simulink model "step4_BatteryModel"  (R2026a)
settings: Solver=daessc  StopTime=82524.31  FixedStep=1e-2  MaxStep=10  MinStep=1e-2  AbsTol=1e-4
undefined symbols (not defined in the file or in its folder): battery_builder_rtmsupport, gcbh
libraries: SHP320_Batteries_lib x8, fl_lib x3, nesl_utility x3, batt_lib x2
(part 2 of 2)

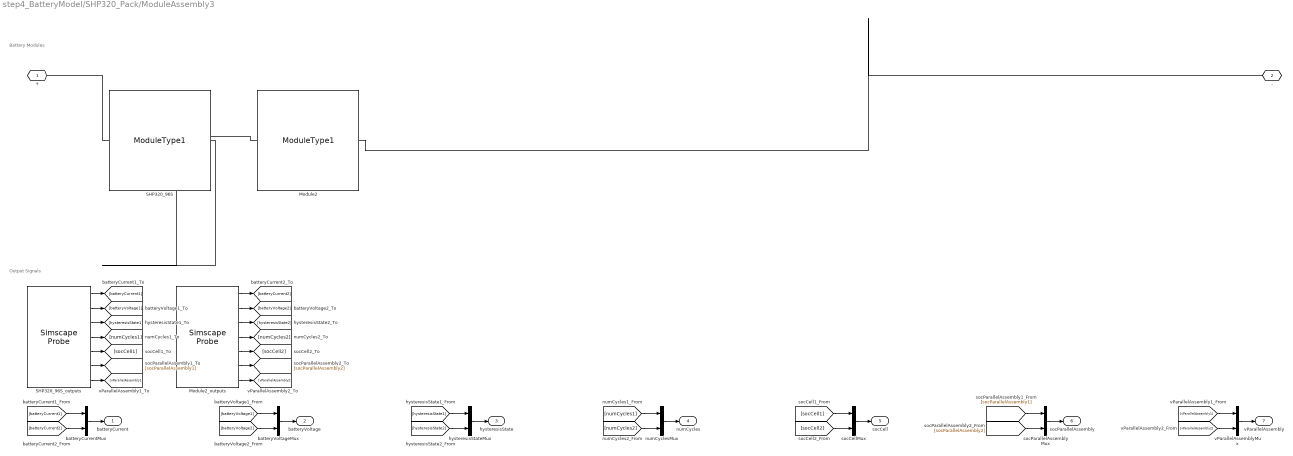
== system step4_BatteryModel/SHP320_Pack/ModuleAssembly3 ==
  note: Output Signals
  note: Battery Modules
  Module2 : SHP320_Batteries_lib/Modules/ModuleType1  BatteryCapacityCell=ModuleType1.BatteryCapacityCell A*hr  ExtrapolationMethodCell=simscape.enum.extrapolation.nearest  SOCBreakpointsCell=ModuleType1.SOCBreakpointsCell  TemperatureBreakpointsCell=ModuleType1.TemperatureBreakpointsCell K  OpenCircuitVoltageThermalCell=ModuleType1.OpenCircuitVoltageThermalCell V  VoltageRangeCell=ModuleType1.VoltageRangeCell V  MaximumHysteresisVoltageThermalCell=ModuleType1.MaximumHysteresisVoltageThermalCell V  InstantaneousHysteresisVoltageThermalCell=ModuleType1.InstantaneousHysteresisVoltageThermalCell V  HysteresisRateThermalCell=ModuleType1.HysteresisRateThermalCell  ResistanceSOCBreakpointsCell=ModuleType1.ResistanceSOCBreakpointsCell  ResistanceTemperatureBreakpointsCell=ModuleType1.ResistanceTemperatureBreakpointsCell K  ChargeR0ThermalCell=ModuleType1.ChargeR0ThermalCell Ohm  DischargeR0ThermalCell=ModuleType1.DischargeR0ThermalCell Ohm  DischargeR1ThermalCell=ModuleType1.DischargeR1ThermalCell Ohm  DischargeTau1ThermalCell=ModuleType1.DischargeTau1ThermalCell s  ChargeR1ThermalCell=ModuleType1.ChargeR1ThermalCell Ohm  ChargeTau1ThermalCell=ModuleType1.ChargeTau1ThermalCell s  DischargeR2ThermalCell=ModuleType1.DischargeR2ThermalCell Ohm  DischargeTau2ThermalCell=ModuleType1.DischargeTau2ThermalCell s  ChargeR2ThermalCell=ModuleType1.ChargeR2ThermalCell Ohm  ChargeTau2ThermalCell=ModuleType1.ChargeTau2ThermalCell s  SimulationTemperatureCell=ModuleType1.SimulationTemperatureCell K  socCell_specify=on  socCell_priority=High  socCell=ModuleAssembly3.Module2.socCell  socCell_nominal_specify=off  socCell_nominal_value=1  socCell_nominal_unit=1  batteryVoltage_specify=on  batteryVoltage_priority=None  batteryVoltage=ModuleAssembly3.Module2.batteryVoltage V  batteryVoltage_nominal_specify=off  batteryVoltage_nominal_value=1  batteryVoltage_nominal_unit=V  batteryCurrent_specify=on  batteryCurrent_priority=None  batteryCurrent=ModuleAssembly3.Module2.batteryCurrent A  batteryCurrent_nominal_specify=off  batteryCurrent_nominal_value=1  batteryCurrent_nominal_unit=A  numCycles_specify=on  numCycles_priority=High  numCycles=ModuleAssembly3.Module2.numCycles  numCycles_nominal_specify=off  numCycles_nominal_value=1  numCycles_nominal_unit=1  hysteresisState_specify=on  hysteresisState_priority=High  hysteresisState=ModuleAssembly3.Module2.hysteresisState  hysteresisState_nominal_specify=off  hysteresisState_nominal_value=1  hysteresisState_nominal_unit=1  vParallelAssembly_specify=on  vParallelAssembly_priority=None  vParallelAssembly=ModuleAssembly3.Module2.vParallelAssembly V  vParallelAssembly_nominal_specify=off  vParallelAssembly_nominal_value=1  vParallelAssembly_nominal_unit=V  socParallelAssembly_specify=on  socParallelAssembly_priority=None  socParallelAssembly=ModuleAssembly3.Module2.socParallelAssembly  socParallelAssembly_nominal_specify=off  socParallelAssembly_nominal_value=1  socParallelAssembly_nominal_unit=1
  Module2_outputs : SimscapeProbe  BoundBlock=72  Variables="{\"batteryCurrent\":{\"Probing\":\"ON\"},\"batteryVoltage\":{\"Probing\":\"ON\"},\"hysteresisState\":{\"Probing\":\"ON\"},\"numCycles\":{\"Probing\":\"ON\"},\"socCell\":{\"Probing\":\"ON\"},\"socParallelAssembly\":{\"Probing\":\"ON\"},\"vParallelAssembly\":{\"Probing\":\"ON\"}}"
  SHP320_96S : SHP320_Batteries_lib/Modules/ModuleType1  BatteryCapacityCell=ModuleType1.BatteryCapacityCell A*hr  ExtrapolationMethodCell=simscape.enum.extrapolation.nearest  SOCBreakpointsCell=ModuleType1.SOCBreakpointsCell  TemperatureBreakpointsCell=ModuleType1.TemperatureBreakpointsCell K  OpenCircuitVoltageThermalCell=ModuleType1.OpenCircuitVoltageThermalCell V  VoltageRangeCell=ModuleType1.VoltageRangeCell V  MaximumHysteresisVoltageThermalCell=ModuleType1.MaximumHysteresisVoltageThermalCell V  InstantaneousHysteresisVoltageThermalCell=ModuleType1.InstantaneousHysteresisVoltageThermalCell V  HysteresisRateThermalCell=ModuleType1.HysteresisRateThermalCell  ResistanceSOCBreakpointsCell=ModuleType1.ResistanceSOCBreakpointsCell  ResistanceTemperatureBreakpointsCell=ModuleType1.ResistanceTemperatureBreakpointsCell K  ChargeR0ThermalCell=ModuleType1.ChargeR0ThermalCell Ohm  DischargeR0ThermalCell=ModuleType1.DischargeR0ThermalCell Ohm  DischargeR1ThermalCell=ModuleType1.DischargeR1ThermalCell Ohm  DischargeTau1ThermalCell=ModuleType1.DischargeTau1ThermalCell s  ChargeR1ThermalCell=ModuleType1.ChargeR1ThermalCell Ohm  ChargeTau1ThermalCell=ModuleType1.ChargeTau1ThermalCell s  DischargeR2ThermalCell=ModuleType1.DischargeR2ThermalCell Ohm  DischargeTau2ThermalCell=ModuleType1.DischargeTau2ThermalCell s  ChargeR2ThermalCell=ModuleType1.ChargeR2ThermalCell Ohm  ChargeTau2ThermalCell=ModuleType1.ChargeTau2ThermalCell s  SimulationTemperatureCell=ModuleType1.SimulationTemperatureCell K  socCell_specify=on  socCell_priority=High  socCell=ModuleAssembly3.SHP320_96S.socCell  socCell_nominal_specify=off  socCell_nominal_value=1  socCell_nominal_unit=1  batteryVoltage_specify=on  batteryVoltage_priority=None  batteryVoltage=ModuleAssembly3.SHP320_96S.batteryVoltage V  batteryVoltage_nominal_specify=off  batteryVoltage_nominal_value=1  batteryVoltage_nominal_unit=V  batteryCurrent_specify=on  batteryCurrent_priority=None  batteryCurrent=ModuleAssembly3.SHP320_96S.batteryCurrent A  batteryCurrent_nominal_specify=off  batteryCurrent_nominal_value=1  batteryCurrent_nominal_unit=A  numCycles_specify=on  numCycles_priority=High  numCycles=ModuleAssembly3.SHP320_96S.numCycles  numCycles_nominal_specify=off  numCycles_nominal_value=1  numCycles_nominal_unit=1  hysteresisState_specify=on  hysteresisState_priority=High  hysteresisState=ModuleAssembly3.SHP320_96S.hysteresisState  hysteresisState_nominal_specify=off  hysteresisState_nominal_value=1  hysteresisState_nominal_unit=1  vParallelAssembly_specify=on  vParallelAssembly_priority=None  vParallelAssembly=ModuleAssembly3.SHP320_96S.vParallelAssembly V  vParallelAssembly_nominal_specify=off  vParallelAssembly_nominal_value=1  vParallelAssembly_nominal_unit=V  socParallelAssembly_specify=on  socParallelAssembly_priority=None  socParallelAssembly=ModuleAssembly3.SHP320_96S.socParallelAssembly  socParallelAssembly_nominal_specify=off  socParallelAssembly_nominal_value=1  socParallelAssembly_nominal_unit=1
  SHP320_96S_outputs : SimscapeProbe  BoundBlock=74  Variables="{\"batteryCurrent\":{\"Probing\":\"ON\"},\"batteryVoltage\":{\"Probing\":\"ON\"},\"hysteresisState\":{\"Probing\":\"ON\"},\"numCycles\":{\"Probing\":\"ON\"},\"socCell\":{\"Probing\":\"ON\"},\"socParallelAssembly\":{\"Probing\":\"ON\"},\"vParallelAssembly\":{\"Probing\":\"ON\"}}"
  batteryCurrentMux : Mux  Inputs=2
  batteryVoltageMux : Mux  Inputs=2
  hysteresisStateMux : Mux  Inputs=2
  numCyclesMux : Mux  Inputs=2
  socCellMux : Mux  Inputs=2
  socParallelAssemblyMux : Mux  Inputs=2
  vParallelAssemblyMux : Mux  Inputs=2
  + : PMIOPort  Side=Left
  - : PMIOPort  Port=2  Side=Right
  batteryCurrent : Outport
  batteryVoltage : Outport  Port=2
  hysteresisState : Outport  Port=3
  numCycles : Outport  Port=4
  socCell : Outport  Port=5
  socParallelAssembly : Outport  Port=6
  vParallelAssembly : Outport  Port=7
  wires:
  [vParallelAssembly2] -> vParallelAssemblyMux/2
  Module2_outputs/7 -> [vParallelAssembly2]
  [socParallelAssembly2] -> socParallelAssemblyMux/2
  Module2_outputs/6 -> [socParallelAssembly2]
  [socCell2] -> socCellMux/2
  Module2_outputs/5 -> [socCell2]
  [numCycles2] -> numCyclesMux/2
  Module2_outputs/4 -> [numCycles2]
  [hysteresisState2] -> hysteresisStateMux/2
  Module2_outputs/3 -> [hysteresisState2]
  [batteryVoltage2] -> batteryVoltageMux/2
  Module2_outputs/2 -> [batteryVoltage2]
  [batteryCurrent2] -> batteryCurrentMux/2
  Module2_outputs/1 -> [batteryCurrent2]
  [vParallelAssembly1] -> vParallelAssemblyMux/1
  vParallelAssemblyMux/1 -> vParallelAssembly/1
  SHP320_96S_outputs/7 -> [vParallelAssembly1]
  [socParallelAssembly1] -> socParallelAssemblyMux/1
  socParallelAssemblyMux/1 -> socParallelAssembly/1
  SHP320_96S_outputs/6 -> [socParallelAssembly1]
  [socCell1] -> socCellMux/1
  socCellMux/1 -> socCell/1
  SHP320_96S_outputs/5 -> [socCell1]
  [numCycles1] -> numCyclesMux/1
  numCyclesMux/1 -> numCycles/1
  SHP320_96S_outputs/4 -> [numCycles1]
  [hysteresisState1] -> hysteresisStateMux/1
  hysteresisStateMux/1 -> hysteresisState/1
  SHP320_96S_outputs/3 -> [hysteresisState1]
  [batteryVoltage1] -> batteryVoltageMux/1
  batteryVoltageMux/1 -> batteryVoltage/1
  SHP320_96S_outputs/2 -> [batteryVoltage1]
  [batteryCurrent1] -> batteryCurrentMux/1
  batteryCurrentMux/1 -> batteryCurrent/1
  SHP320_96S_outputs/1 -> [batteryCurrent1]
  connections:
  Module2/RConn1 -- -/RConn1
  SHP320_96S/LConn1 -- +/RConn1
  Module2/LConn1 -- SHP320_96S/RConn1

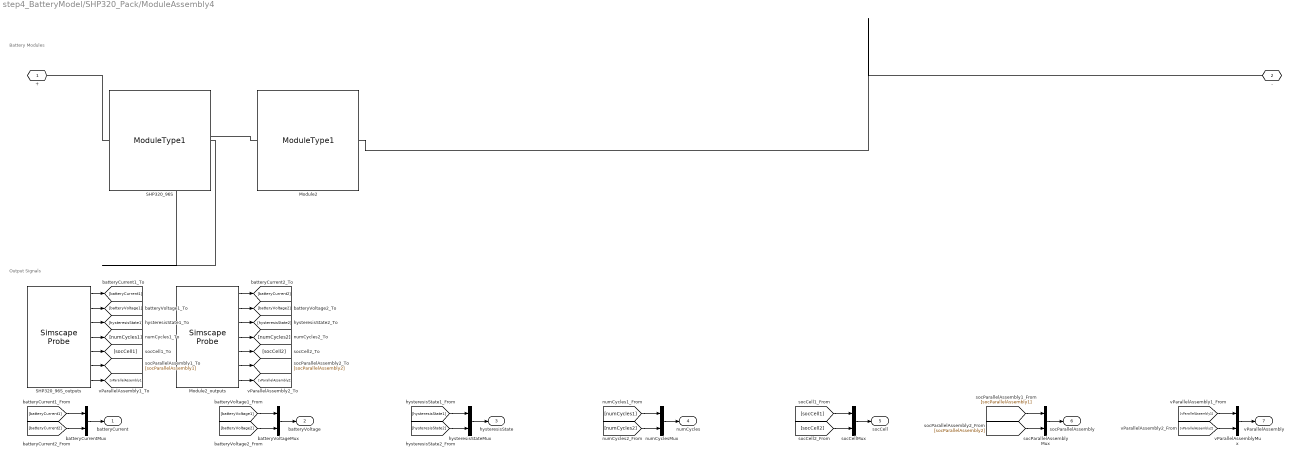
== system step4_BatteryModel/SHP320_Pack/ModuleAssembly4 ==
  note: Output Signals
  note: Battery Modules
  Module2 : SHP320_Batteries_lib/Modules/ModuleType1  BatteryCapacityCell=ModuleType1.BatteryCapacityCell A*hr  ExtrapolationMethodCell=simscape.enum.extrapolation.nearest  SOCBreakpointsCell=ModuleType1.SOCBreakpointsCell  TemperatureBreakpointsCell=ModuleType1.TemperatureBreakpointsCell K  OpenCircuitVoltageThermalCell=ModuleType1.OpenCircuitVoltageThermalCell V  VoltageRangeCell=ModuleType1.VoltageRangeCell V  MaximumHysteresisVoltageThermalCell=ModuleType1.MaximumHysteresisVoltageThermalCell V  InstantaneousHysteresisVoltageThermalCell=ModuleType1.InstantaneousHysteresisVoltageThermalCell V  HysteresisRateThermalCell=ModuleType1.HysteresisRateThermalCell  ResistanceSOCBreakpointsCell=ModuleType1.ResistanceSOCBreakpointsCell  ResistanceTemperatureBreakpointsCell=ModuleType1.ResistanceTemperatureBreakpointsCell K  ChargeR0ThermalCell=ModuleType1.ChargeR0ThermalCell Ohm  DischargeR0ThermalCell=ModuleType1.DischargeR0ThermalCell Ohm  DischargeR1ThermalCell=ModuleType1.DischargeR1ThermalCell Ohm  DischargeTau1ThermalCell=ModuleType1.DischargeTau1ThermalCell s  ChargeR1ThermalCell=ModuleType1.ChargeR1ThermalCell Ohm  ChargeTau1ThermalCell=ModuleType1.ChargeTau1ThermalCell s  DischargeR2ThermalCell=ModuleType1.DischargeR2ThermalCell Ohm  DischargeTau2ThermalCell=ModuleType1.DischargeTau2ThermalCell s  ChargeR2ThermalCell=ModuleType1.ChargeR2ThermalCell Ohm  ChargeTau2ThermalCell=ModuleType1.ChargeTau2ThermalCell s  SimulationTemperatureCell=ModuleType1.SimulationTemperatureCell K  socCell_specify=on  socCell_priority=High  socCell=ModuleAssembly4.Module2.socCell  socCell_nominal_specify=off  socCell_nominal_value=1  socCell_nominal_unit=1  batteryVoltage_specify=on  batteryVoltage_priority=None  batteryVoltage=ModuleAssembly4.Module2.batteryVoltage V  batteryVoltage_nominal_specify=off  batteryVoltage_nominal_value=1  batteryVoltage_nominal_unit=V  batteryCurrent_specify=on  batteryCurrent_priority=None  batteryCurrent=ModuleAssembly4.Module2.batteryCurrent A  batteryCurrent_nominal_specify=off  batteryCurrent_nominal_value=1  batteryCurrent_nominal_unit=A  numCycles_specify=on  numCycles_priority=High  numCycles=ModuleAssembly4.Module2.numCycles  numCycles_nominal_specify=off  numCycles_nominal_value=1  numCycles_nominal_unit=1  hysteresisState_specify=on  hysteresisState_priority=High  hysteresisState=ModuleAssembly4.Module2.hysteresisState  hysteresisState_nominal_specify=off  hysteresisState_nominal_value=1  hysteresisState_nominal_unit=1  vParallelAssembly_specify=on  vParallelAssembly_priority=None  vParallelAssembly=ModuleAssembly4.Module2.vParallelAssembly V  vParallelAssembly_nominal_specify=off  vParallelAssembly_nominal_value=1  vParallelAssembly_nominal_unit=V  socParallelAssembly_specify=on  socParallelAssembly_priority=None  socParallelAssembly=ModuleAssembly4.Module2.socParallelAssembly  socParallelAssembly_nominal_specify=off  socParallelAssembly_nominal_value=1  socParallelAssembly_nominal_unit=1
  Module2_outputs : SimscapeProbe  BoundBlock=123  Variables="{\"batteryCurrent\":{\"Probing\":\"ON\"},\"batteryVoltage\":{\"Probing\":\"ON\"},\"hysteresisState\":{\"Probing\":\"ON\"},\"numCycles\":{\"Probing\":\"ON\"},\"socCell\":{\"Probing\":\"ON\"},\"socParallelAssembly\":{\"Probing\":\"ON\"},\"vParallelAssembly\":{\"Probing\":\"ON\"}}"
  SHP320_96S : SHP320_Batteries_lib/Modules/ModuleType1  BatteryCapacityCell=ModuleType1.BatteryCapacityCell A*hr  ExtrapolationMethodCell=simscape.enum.extrapolation.nearest  SOCBreakpointsCell=ModuleType1.SOCBreakpointsCell  TemperatureBreakpointsCell=ModuleType1.TemperatureBreakpointsCell K  OpenCircuitVoltageThermalCell=ModuleType1.OpenCircuitVoltageThermalCell V  VoltageRangeCell=ModuleType1.VoltageRangeCell V  MaximumHysteresisVoltageThermalCell=ModuleType1.MaximumHysteresisVoltageThermalCell V  InstantaneousHysteresisVoltageThermalCell=ModuleType1.InstantaneousHysteresisVoltageThermalCell V  HysteresisRateThermalCell=ModuleType1.HysteresisRateThermalCell  ResistanceSOCBreakpointsCell=ModuleType1.ResistanceSOCBreakpointsCell  ResistanceTemperatureBreakpointsCell=ModuleType1.ResistanceTemperatureBreakpointsCell K  ChargeR0ThermalCell=ModuleType1.ChargeR0ThermalCell Ohm  DischargeR0ThermalCell=ModuleType1.DischargeR0ThermalCell Ohm  DischargeR1ThermalCell=ModuleType1.DischargeR1ThermalCell Ohm  DischargeTau1ThermalCell=ModuleType1.DischargeTau1ThermalCell s  ChargeR1ThermalCell=ModuleType1.ChargeR1ThermalCell Ohm  ChargeTau1ThermalCell=ModuleType1.ChargeTau1ThermalCell s  DischargeR2ThermalCell=ModuleType1.DischargeR2ThermalCell Ohm  DischargeTau2ThermalCell=ModuleType1.DischargeTau2ThermalCell s  ChargeR2ThermalCell=ModuleType1.ChargeR2ThermalCell Ohm  ChargeTau2ThermalCell=ModuleType1.ChargeTau2ThermalCell s  SimulationTemperatureCell=ModuleType1.SimulationTemperatureCell K  socCell_specify=on  socCell_priority=High  socCell=ModuleAssembly4.SHP320_96S.socCell  socCell_nominal_specify=off  socCell_nominal_value=1  socCell_nominal_unit=1  batteryVoltage_specify=on  batteryVoltage_priority=None  batteryVoltage=ModuleAssembly4.SHP320_96S.batteryVoltage V  batteryVoltage_nominal_specify=off  batteryVoltage_nominal_value=1  batteryVoltage_nominal_unit=V  batteryCurrent_specify=on  batteryCurrent_priority=None  batteryCurrent=ModuleAssembly4.SHP320_96S.batteryCurrent A  batteryCurrent_nominal_specify=off  batteryCurrent_nominal_value=1  batteryCurrent_nominal_unit=A  numCycles_specify=on  numCycles_priority=High  numCycles=ModuleAssembly4.SHP320_96S.numCycles  numCycles_nominal_specify=off  numCycles_nominal_value=1  numCycles_nominal_unit=1  hysteresisState_specify=on  hysteresisState_priority=High  hysteresisState=ModuleAssembly4.SHP320_96S.hysteresisState  hysteresisState_nominal_specify=off  hysteresisState_nominal_value=1  hysteresisState_nominal_unit=1  vParallelAssembly_specify=on  vParallelAssembly_priority=None  vParallelAssembly=ModuleAssembly4.SHP320_96S.vParallelAssembly V  vParallelAssembly_nominal_specify=off  vParallelAssembly_nominal_value=1  vParallelAssembly_nominal_unit=V  socParallelAssembly_specify=on  socParallelAssembly_priority=None  socParallelAssembly=ModuleAssembly4.SHP320_96S.socParallelAssembly  socParallelAssembly_nominal_specify=off  socParallelAssembly_nominal_value=1  socParallelAssembly_nominal_unit=1
  SHP320_96S_outputs : SimscapeProbe  BoundBlock=125  Variables="{\"batteryCurrent\":{\"Probing\":\"ON\"},\"batteryVoltage\":{\"Probing\":\"ON\"},\"hysteresisState\":{\"Probing\":\"ON\"},\"numCycles\":{\"Probing\":\"ON\"},\"socCell\":{\"Probing\":\"ON\"},\"socParallelAssembly\":{\"Probing\":\"ON\"},\"vParallelAssembly\":{\"Probing\":\"ON\"}}"
  batteryCurrentMux : Mux  Inputs=2
  batteryVoltageMux : Mux  Inputs=2
  hysteresisStateMux : Mux  Inputs=2
  numCyclesMux : Mux  Inputs=2
  socCellMux : Mux  Inputs=2
  socParallelAssemblyMux : Mux  Inputs=2
  vParallelAssemblyMux : Mux  Inputs=2
  + : PMIOPort  Side=Left
  - : PMIOPort  Port=2  Side=Right
  batteryCurrent : Outport
  batteryVoltage : Outport  Port=2
  hysteresisState : Outport  Port=3
  numCycles : Outport  Port=4
  socCell : Outport  Port=5
  socParallelAssembly : Outport  Port=6
  vParallelAssembly : Outport  Port=7
  wires:
  [vParallelAssembly2] -> vParallelAssemblyMux/2
  Module2_outputs/7 -> [vParallelAssembly2]
  [socParallelAssembly2] -> socParallelAssemblyMux/2
  Module2_outputs/6 -> [socParallelAssembly2]
  [socCell2] -> socCellMux/2
  Module2_outputs/5 -> [socCell2]
  [numCycles2] -> numCyclesMux/2
  Module2_outputs/4 -> [numCycles2]
  [hysteresisState2] -> hysteresisStateMux/2
  Module2_outputs/3 -> [hysteresisState2]
  [batteryVoltage2] -> batteryVoltageMux/2
  Module2_outputs/2 -> [batteryVoltage2]
  [batteryCurrent2] -> batteryCurrentMux/2
  Module2_outputs/1 -> [batteryCurrent2]
  [vParallelAssembly1] -> vParallelAssemblyMux/1
  vParallelAssemblyMux/1 -> vParallelAssembly/1
  SHP320_96S_outputs/7 -> [vParallelAssembly1]
  [socParallelAssembly1] -> socParallelAssemblyMux/1
  socParallelAssemblyMux/1 -> socParallelAssembly/1
  SHP320_96S_outputs/6 -> [socParallelAssembly1]
  [socCell1] -> socCellMux/1
  socCellMux/1 -> socCell/1
  SHP320_96S_outputs/5 -> [socCell1]
  [numCycles1] -> numCyclesMux/1
  numCyclesMux/1 -> numCycles/1
  SHP320_96S_outputs/4 -> [numCycles1]
  [hysteresisState1] -> hysteresisStateMux/1
  hysteresisStateMux/1 -> hysteresisState/1
  SHP320_96S_outputs/3 -> [hysteresisState1]
  [batteryVoltage1] -> batteryVoltageMux/1
  batteryVoltageMux/1 -> batteryVoltage/1
  SHP320_96S_outputs/2 -> [batteryVoltage1]
  [batteryCurrent1] -> batteryCurrentMux/1
  batteryCurrentMux/1 -> batteryCurrent/1
  SHP320_96S_outputs/1 -> [batteryCurrent1]
  connections:
  Module2/RConn1 -- -/RConn1
  SHP320_96S/LConn1 -- +/RConn1
  Module2/LConn1 -- SHP320_96S/RConn1

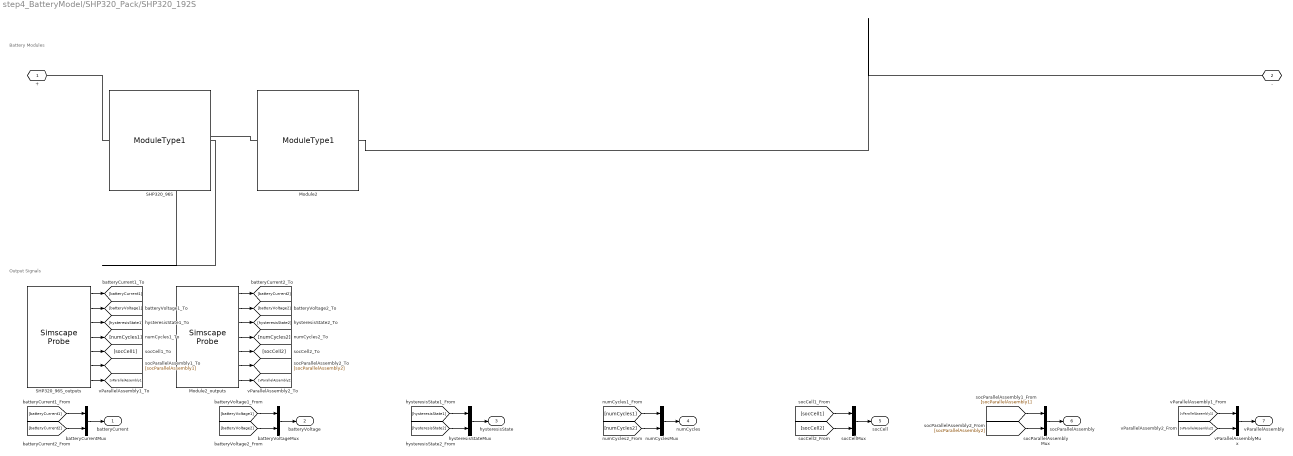
== system step4_BatteryModel/SHP320_Pack/SHP320_192S ==
  note: Output Signals
  note: Battery Modules
  Module2 : SHP320_Batteries_lib/Modules/ModuleType1  BatteryCapacityCell=ModuleType1.BatteryCapacityCell A*hr  ExtrapolationMethodCell=simscape.enum.extrapolation.nearest  SOCBreakpointsCell=ModuleType1.SOCBreakpointsCell  TemperatureBreakpointsCell=ModuleType1.TemperatureBreakpointsCell K  OpenCircuitVoltageThermalCell=ModuleType1.OpenCircuitVoltageThermalCell V  VoltageRangeCell=ModuleType1.VoltageRangeCell V  MaximumHysteresisVoltageThermalCell=ModuleType1.MaximumHysteresisVoltageThermalCell V  InstantaneousHysteresisVoltageThermalCell=ModuleType1.InstantaneousHysteresisVoltageThermalCell V  HysteresisRateThermalCell=ModuleType1.HysteresisRateThermalCell  ResistanceSOCBreakpointsCell=ModuleType1.ResistanceSOCBreakpointsCell  ResistanceTemperatureBreakpointsCell=ModuleType1.ResistanceTemperatureBreakpointsCell K  ChargeR0ThermalCell=ModuleType1.ChargeR0ThermalCell Ohm  DischargeR0ThermalCell=ModuleType1.DischargeR0ThermalCell Ohm  DischargeR1ThermalCell=ModuleType1.DischargeR1ThermalCell Ohm  DischargeTau1ThermalCell=ModuleType1.DischargeTau1ThermalCell s  ChargeR1ThermalCell=ModuleType1.ChargeR1ThermalCell Ohm  ChargeTau1ThermalCell=ModuleType1.ChargeTau1ThermalCell s  DischargeR2ThermalCell=ModuleType1.DischargeR2ThermalCell Ohm  DischargeTau2ThermalCell=ModuleType1.DischargeTau2ThermalCell s  ChargeR2ThermalCell=ModuleType1.ChargeR2ThermalCell Ohm  ChargeTau2ThermalCell=ModuleType1.ChargeTau2ThermalCell s  SimulationTemperatureCell=ModuleType1.SimulationTemperatureCell K  socCell_specify=on  socCell_priority=High  socCell=SHP320_192S.Module2.socCell  socCell_nominal_specify=off  socCell_nominal_value=1  socCell_nominal_unit=1  batteryVoltage_specify=on  batteryVoltage_priority=None  batteryVoltage=SHP320_192S.Module2.batteryVoltage V  batteryVoltage_nominal_specify=off  batteryVoltage_nominal_value=1  batteryVoltage_nominal_unit=V  batteryCurrent_specify=on  batteryCurrent_priority=None  batteryCurrent=SHP320_192S.Module2.batteryCurrent A  batteryCurrent_nominal_specify=off  batteryCurrent_nominal_value=1  batteryCurrent_nominal_unit=A  numCycles_specify=on  numCycles_priority=High  numCycles=SHP320_192S.Module2.numCycles  numCycles_nominal_specify=off  numCycles_nominal_value=1  numCycles_nominal_unit=1  hysteresisState_specify=on  hysteresisState_priority=High  hysteresisState=SHP320_192S.Module2.hysteresisState  hysteresisState_nominal_specify=off  hysteresisState_nominal_value=1  hysteresisState_nominal_unit=1  vParallelAssembly_specify=on  vParallelAssembly_priority=None  vParallelAssembly=SHP320_192S.Module2.vParallelAssembly V  vParallelAssembly_nominal_specify=off  vParallelAssembly_nominal_value=1  vParallelAssembly_nominal_unit=V  socParallelAssembly_specify=on  socParallelAssembly_priority=None  socParallelAssembly=SHP320_192S.Module2.socParallelAssembly  socParallelAssembly_nominal_specify=off  socParallelAssembly_nominal_value=1  socParallelAssembly_nominal_unit=1
  Module2_outputs : SimscapeProbe  BoundBlock=174  Variables="{\"batteryCurrent\":{\"Probing\":\"ON\"},\"batteryVoltage\":{\"Probing\":\"ON\"},\"hysteresisState\":{\"Probing\":\"ON\"},\"numCycles\":{\"Probing\":\"ON\"},\"socCell\":{\"Probing\":\"ON\"},\"socParallelAssembly\":{\"Probing\":\"ON\"},\"vParallelAssembly\":{\"Probing\":\"ON\"}}"
  SHP320_96S : SHP320_Batteries_lib/Modules/ModuleType1  BatteryCapacityCell=ModuleType1.BatteryCapacityCell A*hr  ExtrapolationMethodCell=simscape.enum.extrapolation.nearest  SOCBreakpointsCell=ModuleType1.SOCBreakpointsCell  TemperatureBreakpointsCell=ModuleType1.TemperatureBreakpointsCell K  OpenCircuitVoltageThermalCell=ModuleType1.OpenCircuitVoltageThermalCell V  VoltageRangeCell=ModuleType1.VoltageRangeCell V  MaximumHysteresisVoltageThermalCell=ModuleType1.MaximumHysteresisVoltageThermalCell V  InstantaneousHysteresisVoltageThermalCell=ModuleType1.InstantaneousHysteresisVoltageThermalCell V  HysteresisRateThermalCell=ModuleType1.HysteresisRateThermalCell  ResistanceSOCBreakpointsCell=ModuleType1.ResistanceSOCBreakpointsCell  ResistanceTemperatureBreakpointsCell=ModuleType1.ResistanceTemperatureBreakpointsCell K  ChargeR0ThermalCell=ModuleType1.ChargeR0ThermalCell Ohm  DischargeR0ThermalCell=ModuleType1.DischargeR0ThermalCell Ohm  DischargeR1ThermalCell=ModuleType1.DischargeR1ThermalCell Ohm  DischargeTau1ThermalCell=ModuleType1.DischargeTau1ThermalCell s  ChargeR1ThermalCell=ModuleType1.ChargeR1ThermalCell Ohm  ChargeTau1ThermalCell=ModuleType1.ChargeTau1ThermalCell s  DischargeR2ThermalCell=ModuleType1.DischargeR2ThermalCell Ohm  DischargeTau2ThermalCell=ModuleType1.DischargeTau2ThermalCell s  ChargeR2ThermalCell=ModuleType1.ChargeR2ThermalCell Ohm  ChargeTau2ThermalCell=ModuleType1.ChargeTau2ThermalCell s  SimulationTemperatureCell=ModuleType1.SimulationTemperatureCell K  socCell_specify=on  socCell_priority=High  socCell=SHP320_192S.SHP320_96S.socCell  socCell_nominal_specify=off  socCell_nominal_value=1  socCell_nominal_unit=1  batteryVoltage_specify=on  batteryVoltage_priority=None  batteryVoltage=SHP320_192S.SHP320_96S.batteryVoltage V  batteryVoltage_nominal_specify=off  batteryVoltage_nominal_value=1  batteryVoltage_nominal_unit=V  batteryCurrent_specify=on  batteryCurrent_priority=None  batteryCurrent=SHP320_192S.SHP320_96S.batteryCurrent A  batteryCurrent_nominal_specify=off  batteryCurrent_nominal_value=1  batteryCurrent_nominal_unit=A  numCycles_specify=on  numCycles_priority=High  numCycles=SHP320_192S.SHP320_96S.numCycles  numCycles_nominal_specify=off  numCycles_nominal_value=1  numCycles_nominal_unit=1  hysteresisState_specify=on  hysteresisState_priority=High  hysteresisState=SHP320_192S.SHP320_96S.hysteresisState  hysteresisState_nominal_specify=off  hysteresisState_nominal_value=1  hysteresisState_nominal_unit=1  vParallelAssembly_specify=on  vParallelAssembly_priority=None  vParallelAssembly=SHP320_192S.SHP320_96S.vParallelAssembly V  vParallelAssembly_nominal_specify=off  vParallelAssembly_nominal_value=1  vParallelAssembly_nominal_unit=V  socParallelAssembly_specify=on  socParallelAssembly_priority=None  socParallelAssembly=SHP320_192S.SHP320_96S.socParallelAssembly  socParallelAssembly_nominal_specify=off  socParallelAssembly_nominal_value=1  socParallelAssembly_nominal_unit=1
  SHP320_96S_outputs : SimscapeProbe  BoundBlock=176  Variables="{\"batteryCurrent\":{\"Probing\":\"ON\"},\"batteryVoltage\":{\"Probing\":\"ON\"},\"hysteresisState\":{\"Probing\":\"ON\"},\"numCycles\":{\"Probing\":\"ON\"},\"socCell\":{\"Probing\":\"ON\"},\"socParallelAssembly\":{\"Probing\":\"ON\"},\"vParallelAssembly\":{\"Probing\":\"ON\"}}"
  batteryCurrentMux : Mux  Inputs=2
  batteryVoltageMux : Mux  Inputs=2
  hysteresisStateMux : Mux  Inputs=2
  numCyclesMux : Mux  Inputs=2
  socCellMux : Mux  Inputs=2
  socParallelAssemblyMux : Mux  Inputs=2
  vParallelAssemblyMux : Mux  Inputs=2
  + : PMIOPort  Side=Left
  - : PMIOPort  Port=2  Side=Right
  batteryCurrent : Outport
  batteryVoltage : Outport  Port=2
  hysteresisState : Outport  Port=3
  numCycles : Outport  Port=4
  socCell : Outport  Port=5
  socParallelAssembly : Outport  Port=6
  vParallelAssembly : Outport  Port=7
  wires:
  [vParallelAssembly2] -> vParallelAssemblyMux/2
  Module2_outputs/7 -> [vParallelAssembly2]
  [socParallelAssembly2] -> socParallelAssemblyMux/2
  Module2_outputs/6 -> [socParallelAssembly2]
  [socCell2] -> socCellMux/2
  Module2_outputs/5 -> [socCell2]
  [numCycles2] -> numCyclesMux/2
  Module2_outputs/4 -> [numCycles2]
  [hysteresisState2] -> hysteresisStateMux/2
  Module2_outputs/3 -> [hysteresisState2]
  [batteryVoltage2] -> batteryVoltageMux/2
  Module2_outputs/2 -> [batteryVoltage2]
  [batteryCurrent2] -> batteryCurrentMux/2
  Module2_outputs/1 -> [batteryCurrent2]
  [vParallelAssembly1] -> vParallelAssemblyMux/1
  vParallelAssemblyMux/1 -> vParallelAssembly/1
  SHP320_96S_outputs/7 -> [vParallelAssembly1]
  [socParallelAssembly1] -> socParallelAssemblyMux/1
  socParallelAssemblyMux/1 -> socParallelAssembly/1
  SHP320_96S_outputs/6 -> [socParallelAssembly1]
  [socCell1] -> socCellMux/1
  socCellMux/1 -> socCell/1
  SHP320_96S_outputs/5 -> [socCell1]
  [numCycles1] -> numCyclesMux/1
  numCyclesMux/1 -> numCycles/1
  SHP320_96S_outputs/4 -> [numCycles1]
  [hysteresisState1] -> hysteresisStateMux/1
  hysteresisStateMux/1 -> hysteresisState/1
  SHP320_96S_outputs/3 -> [hysteresisState1]
  [batteryVoltage1] -> batteryVoltageMux/1
  batteryVoltageMux/1 -> batteryVoltage/1
  SHP320_96S_outputs/2 -> [batteryVoltage1]
  [batteryCurrent1] -> batteryCurrentMux/1
  batteryCurrentMux/1 -> batteryCurrent/1
  SHP320_96S_outputs/1 -> [batteryCurrent1]
  connections:
  Module2/RConn1 -- -/RConn1
  SHP320_96S/LConn1 -- +/RConn1
  Module2/LConn1 -- SHP320_96S/RConn1
